simulink model "Old Subsystem"  (R2021a)
settings: Solver=VariableStepAuto  StartTime=0.0  StopTime=10.0  RelTol=1e-3
undefined symbols (not defined in the file): AirSpeed, Gravity, Height, RollAngle, WindDown, WindEast, WindNorth
libraries: uavalgslib x1
settings DebuggingCC: UnconnectedInputMsg=none  UnconnectedOutputMsg=none  UnconnectedLineMsg=none
settings ModelReferenceCC: EnableRefExpFcnMdlSchedulingChecks=off
settings RTWCC: Description=Generic Real-Time Target  GPUComputeCapability=5.0  DLArmComputeVersion=20.02.1

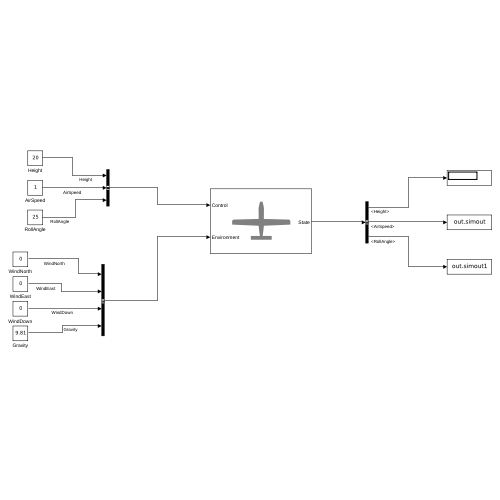
[thumbnail: Simulink's stored preview of the top-level diagram]
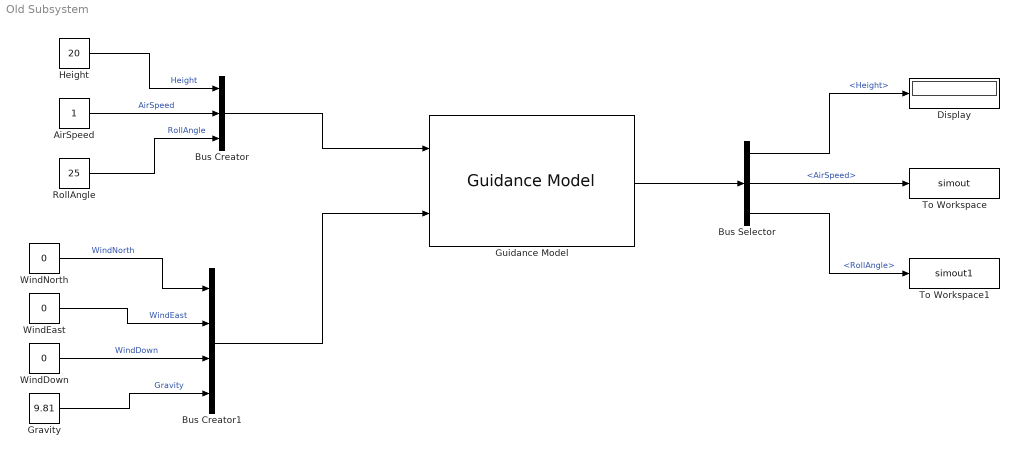
== system Old Subsystem ==
  AirSpeed : Constant
  Bus Creator : BusCreator  Inputs=Height,AirSpeed,RollAngle  OutDataTypeStr=Bus: FixedWingGuidanceControlBus  NonVirtualBus=on
  Bus Creator1 : BusCreator  Inputs=WindNorth,WindEast,WindDown,Gravity  OutDataTypeStr=Bus: FixedWingGuidanceEnvironmentBus  NonVirtualBus=on
  Bus Selector : BusSelector  OutputSignals=Height,AirSpeed,RollAngle
  Display : Display
  Gravity : Constant  Value=9.81
  Guidance Model : uavalgslib/Guidance Model  ModelType=FixedWingGuidance  SpecifiedDataType=double  SimulateUsing=Interpreted execution  InitialWorldPositionMultirotor=[0; 0; 0]  InitialWorldVelocityMultirotor=[0; 0; 0]  InitialEulerZYXMultirotor=[0; 0; 0]  InitialBodyAngularRateRPYMultirotor=[0; 0; 0]  InitialThrustMultirotor=0  InitialNorthFixedWing=0  InitialEastFixedWing=0  InitialHeightFixedWing=0  InitialAirSpeedFixedWing=0  InitialHeadingAngleFixedWing=0  InitialFlightPathAngleFixedWing=0  InitialRollAngleFixedWing=0  InitialRollAngleRateFixedWing=0  PDRollMultirotor=[3402.97,116.67]  PDPitchMultirotor=[3402.97, 116.67]  PYawRateMultirotor=1950  PThrustMultirotor=3900  MassMultirotor=0.1  PHeightFixedWing=3.9  PHeadingAngleFixedWing=3.9  PFlightPathAngleFixedWing=39  PDRollFixedWing=[3402.97, 116.67]  PAirSpeedFixedWing=1  FlightPathAngleLimitsFixedWing=[-pi/2, pi/2]  StateBusName='FixedWingGuidanceStateBus'  ControlBusName='FixedWingGuidanceControlBus'  EnvironmentBusName='FixedWingGuidanceEnvironmentBus'  DataType=double
  Height : Constant  Value=20
  RollAngle : Constant  Value=25
  To Workspace : ToWorkspace  VariableName=simout  SaveFormat=Timeseries  SampleTime=-1
  To Workspace1 : ToWorkspace  VariableName=simout1  SaveFormat=Timeseries  SampleTime=-1
  WindDown : Constant  Value=0
  WindEast : Constant  Value=0
  WindNorth : Constant  Value=0
  wires:
  Height/1 -> Bus Creator/1  "Height"
  AirSpeed/1 -> Bus Creator/2  "AirSpeed"
  RollAngle/1 -> Bus Creator/3  "RollAngle"
  Bus Creator/1 -> Guidance Model/1
  WindNorth/1 -> Bus Creator1/1  "WindNorth"
  WindEast/1 -> Bus Creator1/2  "WindEast"
  WindDown/1 -> Bus Creator1/3  "WindDown"
  Gravity/1 -> Bus Creator1/4  "Gravity"
  Bus Creator1/1 -> Guidance Model/2
  Guidance Model/1 -> Bus Selector/1
  Bus Selector/2 -> To Workspace/1  "<AirSpeed>"
  Bus Selector/1 -> Display/1  "<Height>"
  Bus Selector/3 -> To Workspace1/1  "<RollAngle>"
